simulink subsystem "VorsteuerungMotor"  (R2020a)
settings: Solver=VariableStepAuto  StartTime=0.0  StopTime=10.0  RelTol=1e-3
model mask{MotorGain=0}
  mask prompts: MotorGain "Static Motor Gain"
settings Model: Creator=Tobias  LastModifiedBy=Tobias

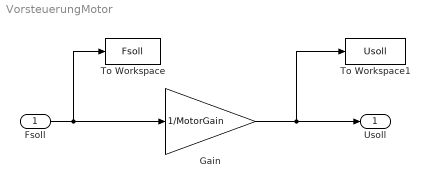
== system VorsteuerungMotor ==
  Fsoll : Inport
  Gain : Gain  Gain=1/MotorGain
  To Workspace : ToWorkspace  VariableName=Fsoll  SaveFormat=Timeseries  SampleTime=-1
  To Workspace1 : ToWorkspace  VariableName=Usoll  SaveFormat=Timeseries  SampleTime=-1
  Usoll : Outport
  wires:
  Gain/1 -> Usoll/1, To Workspace1/1
  Fsoll/1 -> To Workspace/1, Gain/1
